simulink model "controlado"  (R2020a)
settings: Solver=VariableStepAuto  StartTime=0.0  StopTime=30  RelTol=1e-3
values from neighbouring files (symbols this model uses):
  A = [0 0 1 0; 0 0 0 1; 0 0 -den_p(2) 0; 0 -den_a(3) 0 -den_a(2)]    [controles.m]
  B = [0; num_a(2); num_p(3); k_techo*num_a(2)*(num_a(3)/num_a(2))]    [controles.m]
  C = [1 0 0 0; 0 1 0 0]    [controles.m]
  K = K2    [controles.m]
  Ki = Ki2    [controles.m]
libraries: simulink x1
settings Model: Creator=Usuario  LastModifiedBy=Usuario

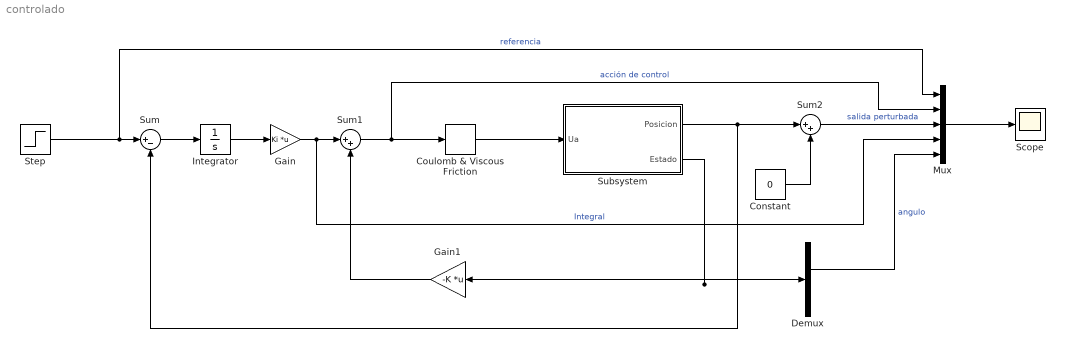
== system controlado ==
  Constant : Constant  Value=0
  Coulomb & Viscous Friction : simulink/Discontinuities/Coulomb & Viscous Friction  offset=[0.4]  gain=1
  Demux : Demux
  Gain : Gain  Gain=Ki  Multiplication=Matrix(K*u)
  Gain1 : Gain  Gain=-K  Multiplication=Matrix(K*u)
  Integrator : Integrator
  Mux : Mux  Inputs=5
  Scope : Scope
  Step : Step  After=0.5  SampleTime=0
  Subsystem : Subsystem
  Sum : Sum  Inputs=|+-
  Sum1 : Sum  Inputs=|++
  Sum2 : Sum  Inputs=|++
  wires:
  Step/1 -> Mux/1, Sum/1  "referencia"
  Sum/1 -> Integrator/1
  Integrator/1 -> Gain/1
  Gain/1 -> Mux/4, Sum1/1  "Integral"
  Sum1/1 -> Mux/2, Coulomb & Viscous Friction/1  "acción de control"
  Coulomb & Viscous Friction/1 -> Subsystem/1(Ua)
  Subsystem/2(Estado) -> Gain1/1, Demux/1
  Gain1/1 -> Sum1/2
  Subsystem/1(Posicion) -> Sum2/1, Sum/2
  Sum2/1 -> Mux/3  "salida perturbada"
  Mux/1 -> Scope/1
  Constant/1 -> Sum2/2
  Demux/2 -> Mux/5  "angulo"

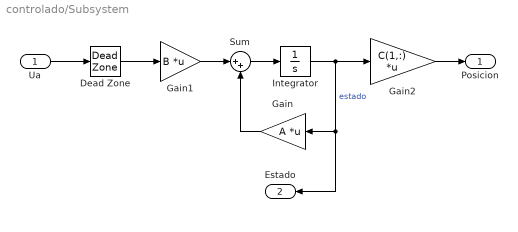
== system controlado/Subsystem ==
  Ua : Inport
  Dead Zone : DeadZone  UpperValue=0.6  SaturateOnIntegerOverflow=on
  Gain : Gain  Gain=A  Multiplication=Matrix(K*u)
  Gain1 : Gain  Gain=B  Multiplication=Matrix(K*u)
  Gain2 : Gain  Gain=C(1,:)  Multiplication=Matrix(K*u)
  Integrator : Integrator
  Sum : Sum  Inputs=|++
  Posicion : Outport
  Estado : Outport  Port=2
  wires:
  Ua/1 -> Dead Zone/1
  Dead Zone/1 -> Gain1/1
  Gain1/1 -> Sum/1
  Sum/1 -> Integrator/1
  Gain/1 -> Sum/2
  Integrator/1 -> Estado/1, Gain/1, Gain2/1  "estado"
  Gain2/1 -> Posicion/1
